simulink model "fmtx_datafm_image_audio"  (R2014b)
settings: Solver=ode45  StartTime=0.0  StopTime=1000*100/3e3  RelTol=1e-3
PreLoadFcn:
  | %%%%%%%%%%%%%%%%%%%%%%%%%%%%%%%%%%%%%%%%%%%%%%%%%%%%%%%%%%%%%%%%%%%%%%%%%%%
  | % check to see if Simulink library folder is missing from the MATLAB path %
  | %%%%%%%%%%%%%%%%%%%%%%%%%%%%%%%%%%%%%%%%%%%%%%%%%%%%%%%%%%%%%%%%%%%%%%%%%%%
  | if isempty(strfind(path, 'rtlsdr_book_library'))
  | 
  |     % create error window
  |     fig_error = figure(...
  |         'Name', 'Error: RTL-SDR Book Library',...
  |         'Toolbar','none',...
  |         'MenuBar','none',...
  |         'NumberTitle','off',...
  |         'Resize','off',...
  |         'WindowStyle','modal');
  |     fig_error.Position(3) = 600;
  |     fig_error.Position(4) = 150;
  |     fig_axes = axes(...
  |         'Parent',fig_error,...
  |         'Position',[0,0,1,1],...
  |         'visible','off');
  |     % error message
  |     t_title = text(.05,.8,...
  |         'MISSING DIRECTORIES',...
  |         'FontSize',11.5);
  |     t_body = text(.075,.6,...
  |         [{'Simulink cannot find the  \it{<root>}\rm / \it{rtlsdr\_book\_library}\rm  folder in the \it{MATLAB Path}\rm.'},...
  |         {'Please set the MATLAB path following the instructions given in Exercise 2.4.'}],...
  |         'FontSize',10.5);
  |     % buttons
  |     btn_path = uicontrol(...
  |         'Parent',fig_error,...
  |         'String','Set Path Now',...
  |         'FontSize',10,...
  |         'Callback', 'pathtool; close(fig_error);',...
  |         'Position', [fig_error.Position(3)/2-210, 30, 200, 30]);
  |     btn_abort = uicontrol(...
  |         'Parent',fig_error,...
  |         'String','No thanks',...
  |         'FontSize',10,...
  |         'Callback', 'close(fig_error); abort=1;',...
  |         'Position', [fig_error.Position(3)/2+10, 30, 200, 30]);
  | 
  |     % pause to allow user to interact with error box
  |     uiwait(fig_error);
  | 
  |     % abort simulation
  |     try
  |         if abort==1
  |             set_param(gcs, 'SimulationCommand', 'stop');
  |         end
  |     end
  | 
  |     % if user has set path, allow diagram to be updated
  |     if ~exist('abort','var')
  |         % create error window
  |         fig_update = figure(...
  |             'Name', 'Update Diagram',...
  |             'Toolbar','none',...
  |             'MenuBar','none',...
  |             'NumberTitle','off',...
  |             'Resize','off');
  |         fig_update.Position(3) = 400;
  |         fig_update.Position(4) = 120;
  |         fig_axes = axes(...
  |             'Parent',fig_update,...
  |             'Position',[0,0,1,1],...
  |             'visible','off');
  |         % instruction message
  |         t_body = text(.075,.7,...
  |             'Once you have set the path, update the block diagram',...
  |             'FontSize',10.5);
  |         % button
  |         btn_update = uicontrol(...
  |             'Parent',fig_update,...
  |             'String','Update Block Diagram',...
  |             'FontSize',10,...
  |             'Callback', 'set_param(gcs,''SimulationCommand'',''update''); close(gcf)',...
  |             'Position', [fig_update.Position(3)/2-100, 30, 200, 30]);
  |     end
  | 
  |     % clear error components
  |     clear('fig_error','fig_update','fig_axes','t_title','t_body','btn_path','btn_abort','btn_update','abort');
  | 
  | end
  | %%%%%%%%%%%%%%%%%%%%%%%%%%%%%%%%%%%%%%%%%%%%%%%%%%%%%%%%%%%%%%%%%%%%%%%%%%%
undefined symbols (not defined in the file): dfilt, fdesignblkfcn, gcbh
libraries: dspvision x2, rtlsdr_book_library x2, dsparch4 x1, dspsrcs4 x1
CloseFcn:
  | closefcn_model;
Description:
  | Software, Simulation Examples and Design Exercises Licence Agreement
  | 
  | This license agreement refers to the simulation examples, design exercises and files,
  | and associated software MATLAB and Simulink resources that accompany the book:
  | 
  |      Title: Software Defined Radio using MATLAB & Simulink and the RTL-SDR
  |      Published by Strathclyde Academic Media, 2015
  |      Authored by Robert W. Stewart, Kenneth W. Barlee, Dale S.W. Atkinson,
  |      and Louise H. Crockett
  | 
  | and made available as a download from, www.desktopSDR.com or variously acquired
  | by other means such as via USB storage, cloud storage, disk or any other electronic
  | or optical or magnetic storage mechanism. These files and associated software may
  | be used subject to the terms of agreement of the conditions below:
  | 
  |     Copyright © 2015 Robert W. Stewart, Kenneth W. Barlee, Dale S.W. Atkinson,
  |     and Louise H. Crockett
  |     All rights reserved.
  | 
  | Redistribution and use in source and binary forms, with or without modification, are
  | permitted provided that the following conditions are met:
  | 
  |    1.  Redistributions of source code must retain the above copyright notice, this list of
  |         conditions and the following disclaimer.
  | 
  |    2.  Redistributions in binary form must reproduce the above copyright notice, this
  |         list of conditions and the following disclaimer in the documentation and/or other
  |         materials provided with the distribution.
  | 
  |    3.  Neither the name of the copyright holder nor the names of its contributors may
  |         be used to endorse or promote products derived from this software without
  |         specific prior written permission.
  | 
  |    4.  In all cases, the software is, and all modifications and derivatives of the
  |         software shall be, licensed to you solely for use in conjunction with The
  |         MathWorks, Inc. products and service offerings.
  | 
  | THIS SOFTWARE IS PROVIDED BY THE COPYRIGHT HOLDERS AND CONTRIBUTORS
  | "AS IS" AND ANY EXPRESS OR IMPLIED WARRANTIES, INCLUDING, BUT NOT LIMITED
  | TO, THE IMPLIED WARRANTIES OF MERCHANTABILITY AND FITNESS FOR A
  | PARTICULAR PURPOSE ARE DISCLAIMED. IN NO EVENT SHALL THE COPYRIGHT
  | HOLDER OR CONTRIBUTORS BE LIABLE FOR ANY DIRECT, INDIRECT, INCIDENTAL,
  | SPECIAL, EXEMPLARY, OR CONSEQUENTIAL DAMAGES (INCLUDING, BUT NOT
  | LIMITED TO, PROCUREMENT OF SUBSTITUTE GOODS OR SERVICES; LOSS OF USE,
  | DATA, OR PROFITS; OR BUSINESS INTERRUPTION) HOWEVER CAUSED AND ON ANY
  | THEORY OF LIABILITY, WHETHER IN CONTRACT, STRICT LIABILITY, OR TORT
  | (INCLUDING NEGLIGENCE OR OTHERWISE) ARISING IN ANY WAY OUT OF THE USE
  | OF THIS SOFTWARE, EVEN IF ADVISED OF THE POSSIBILITY OF SUCH DAMAGE.
  | 
  | 
  | Audio Tracks used in Simulations Examples and Design Exercises
  | 
  | The music and vocal files used within the Examples files and software within the book
  | were variously written, arranged, performed, recorded and produced by Garrey Rice,
  | Adam Struth, Jamie Struth, Iain Thistlethwaite and also Marshall Craigmyle who
  | collectively, and individually where appropriate, assert and retain all of their copyright,
  | performance and artistic rights. Permission to use and reproduce this music is
  | granted for all purposes associated with MATLAB and Simulink software and the
  | simulation examples and design exercises files that accompany this book. Requests to
  | use the music for any other purpose should be directed to: info@desktopSDR.com.
  | For information on music track names, full credits, and links to the musicians please
  | refer to www.desktopSDR.com/more/audio.
settings Model: Creator=desktopSDR Team  LastModifiedBy=desktopSDR Team
settings DataIOCC: LimitDataPoints=off  SaveOutput=off  SignalLogging=off  SaveTime=off

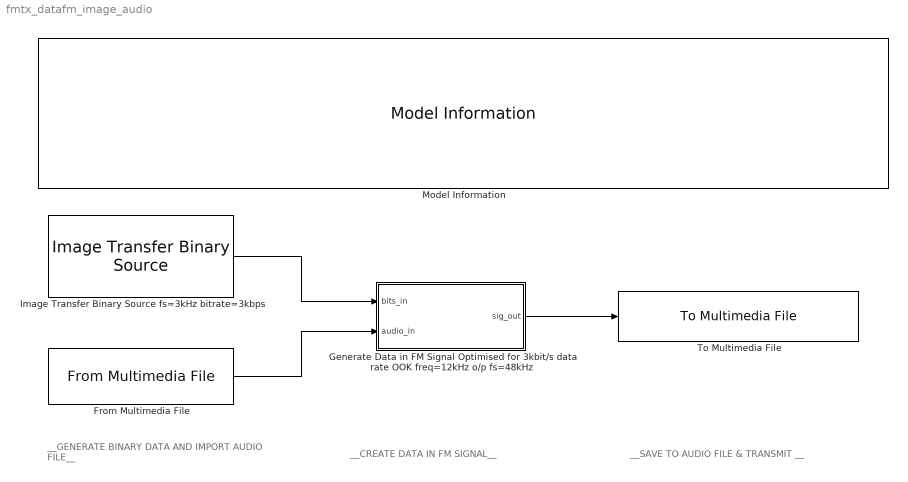
== system fmtx_datafm_image_audio ==
  note: __CREATE DATA IN FM SIGNAL__
  note: __SAVE TO AUDIO FILE & TRANSMIT __
  note: __GENERATE BINARY DATA
      | AND IMPORT AUDIO FILE__
  From Multimedia File : dspvision/From Multimedia File  inputFilename=..\..\audio_sources\music3_mono48kHz.wav  loop=on  numPlays=inf  outputStreams=Audio only  videoDataType=single  audioDataType=double  inheritSampleTime=on  userDefinedSampleTime=1/30  noAudioOutput=off  isIntensityVideo=off  fourcc=RGB  colorVideoFormat=Separate color signals  outputEOF=off  dataOrg=Column-major  audioFrameSize=1024  computeAudioFrameSize=off  outSamplingMode=Frame based
  Generate Data in FM Signal Optimised for 3kbit/s data rate OOK freq=12kHz o/p fs=48kHz : Subsystem
  Image Transfer Binary Source fs=3kHz bitrate=3kbps : rtlsdr_book_library/Data Comms Sources and Sinks/Image Transfer Binary Source  filename=image1.mat  fs=3e3
  Model Information : rtlsdr_book_library/Additional Tools/Model Information/Model Information
  To Multimedia File : dspvision/To Multimedia File  outputFilename=fmtx_datafm_image1_audio.wav  streamSelection=Audio only  videoCompressor=None (uncompressed)  audioCompressor=None (uncompressed)  imagePorts=Separate color signals  fileType=WAV  audioDatatype=16-bit integer  fourcc=RGB  videoQuality=75  mj2000CompFactor=10
  wires:
  Generate Data in FM Signal Optimised for 3kbit/s data rate OOK freq=12kHz o/p fs=48kHz/1(sig_out) -> To Multimedia File/1
  From Multimedia File/1 -> Generate Data in FM Signal Optimised for 3kbit/s data rate OOK freq=12kHz o/p fs=48kHz/2(audio_in)
  Image Transfer Binary Source fs=3kHz bitrate=3kbps/1 -> Generate Data in FM Signal Optimised for 3kbit/s data rate OOK freq=12kHz o/p fs=48kHz/1(bits_in)

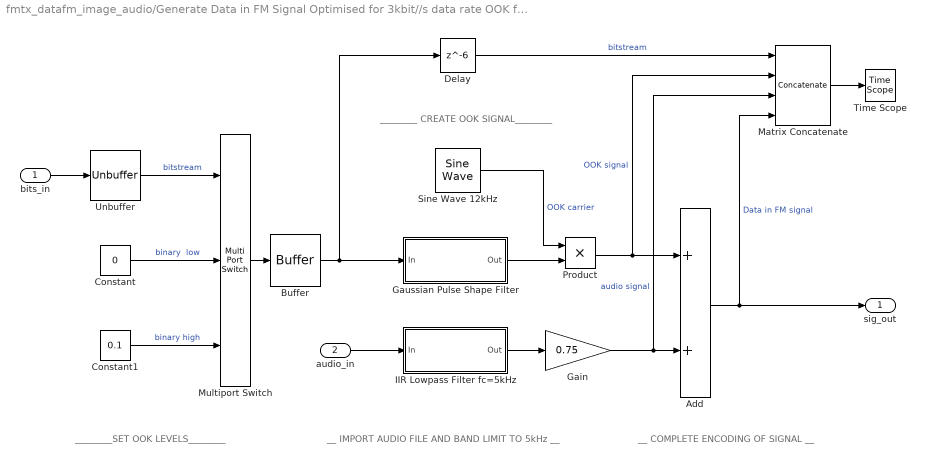
== system fmtx_datafm_image_audio/Generate Data in FM Signal Optimised for 3kbit//s data rate OOK freq=12kHz o//p fs=48kHz ==
  note: __ IMPORT AUDIO FILE AND BAND LIMIT TO 5kHz __
  note: __ COMPLETE ENCODING OF SIGNAL __
  note: ________ CREATE OOK SIGNAL________
  note: ________SET OOK LEVELS________
  bits_in : Inport
  audio_in : Inport  Port=2
  Add : Sum
  Buffer : Buffer  N=1024  TreatMby1Signals=One channel
  Constant : Constant  Value=0  SampleTime=1/48e3
  Constant1 : Constant  Value=0.1  SampleTime=1/48e3
  Delay : Delay  DelayLength=6  InputProcessing=Columns as channels (frame based)
  Gain : Gain  Gain=0.75
  Gaussian Pulse Shape Filter : Subsystem  DialogController=fdesignblkfcn  InitFcn=fdesignblkfcn(gcbh, {'InitFcn'});  mask(Pulse Shaping Filter){}
      mask help: Design a Pulse Shaping Filter
      settings: CopyFcn=fdesignblkfcn(gcbh, {'CopyFcn'});
      mask Help: helpview(mapfilelocation('dsp'), 'dsppulseshapingfilter');
      mask Display: disp('Pulse Shaping');
  IIR Lowpass Filter fc=5kHz : Subsystem  DialogController=fdesignblkfcn  InitFcn=fdesignblkfcn(gcbh, {'InitFcn'});  mask(Lowpass Filter){}
      mask help: Design a lowpass filter
      settings: CopyFcn=fdesignblkfcn(gcbh, {'CopyFcn'});
      mask Help: helpview(mapfilelocation('dsp'), 'dsplowpassfilter');
      mask Display: disp('Lowpass')
  Matrix Concatenate : Concatenate  NumInputs=4  Mode=Multidimensional array  ConcatenateDimension=2
  Multiport Switch : MultiPortSwitch  DataPortOrder=Specify indices  Inputs=2  DataPortIndices={0,1}
  Product : Product
  Sine Wave 12kHz : dspsrcs4/Sine Wave  Amplitude=1  Frequency=12e3  Phase=pi/6  SampleMode=Discrete  OutComplex=Real  CompMethod=Trigonometric fcn  TableSize=Speed  SampleTime=1/48e3  SamplesPerFrame=1024  ResetState=Restart at time zero  dataType=double  wordLen=16  udDataType=sfix(16)  fracBitsMode=Best precision  numFracBits=15  OutDataTypeStr=double  LastOutDataTypeStr=double
  Time Scope : TimeScope  StartFcn=startfcn_time_scope  DefaultConfigurationName=spbscopes.TimeScopeBlockCfg
  Unbuffer : Unbuffer  SampleBasedProcessing=Same as frame based
  sig_out : Outport
  wires:
  bits_in/1 -> Unbuffer/1
  audio_in/1 -> IIR Lowpass Filter fc=5kHz/1(In)
  Constant1/1 -> Multiport Switch/3  "binary high"
  Constant/1 -> Multiport Switch/2  "binary  low"
  Matrix Concatenate/1 -> Time Scope/1
  IIR Lowpass Filter fc=5kHz/1(Out) -> Gain/1
  Gain/1 -> Matrix Concatenate/3, Add/2  "audio signal"
  Unbuffer/1 -> Multiport Switch/1  "bitstream"
  Sine Wave 12kHz/1 -> Product/1  "OOK carrier"
  Buffer/1 -> Delay/1, Gaussian Pulse Shape Filter/1(In)
  Gaussian Pulse Shape Filter/1(Out) -> Product/2
  Product/1 -> Matrix Concatenate/2, Add/1  "OOK signal"
  Multiport Switch/1 -> Buffer/1
  Add/1 -> Matrix Concatenate/4, sig_out/1  "Data in FM signal"
  Delay/1 -> Matrix Concatenate/1  "bitstream"

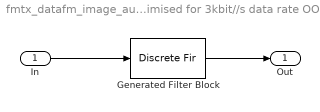
== system fmtx_datafm_image_audio/Generate Data in FM Signal Optimised for 3kbit//s data rate OOK freq=12kHz o//p fs=48kHz/Gaussian Pulse Shape Filter ==
  In : Inport
  Generated Filter Block : DiscreteFir  Tag=BlockMethodSubSystem  Coefficients=[0.011762699801536648 0.02574058949880206 0.048853030996808648 0.080412967456829659 0.11479479958541473 0.14212808000788887 0.15261566530543869 0.14212808000788887 0.11479479958541473 0.080412967456829659 0.048853030996808648 0.02574058949880206 0.011762699801536648]  InputProcessing=Columns as channels (frame based)
  Out : Outport
  wires:
  In/1 -> Generated Filter Block/1
  Generated Filter Block/1 -> Out/1

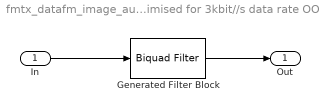
== system fmtx_datafm_image_audio/Generate Data in FM Signal Optimised for 3kbit//s data rate OOK freq=12kHz o//p fs=48kHz/IIR Lowpass Filter fc=5kHz ==
  In : Inport
  Generated Filter Block : dsparch4/Biquad Filter  Tag=BlockMethodSubSystem  IIRFiltStruct=Direct form II  CoeffSource=Specify via dialog  BiQuadCoeffs=[0.042969561565618077 0.085939123131236153 0.042969561565618077 1 -1.555657758639478 0.87862894950711246;0.061935778665187145 0.12387155733037429 0.061935778665187145 1 -1.4205854439157277 0.71551417743867618;0.076267506257963871 0.15253501251592774 0.076267506257963871 1 -1.3129466799361755 0.58552845469333503;0.086601072542009133 0.17320214508401827 0.086601072542009133 1 -1.2285300304649582 0.48358600582481348;0.093330556989539987 0.18666111397907997 0.093330556989539987 1 -1.163928907888546 0.40557299919227274;0.096444753467057845 0.19288950693411569 0.096444753467057845 1 -1.1165183760349042 0.34831953379659664;0.093941235402774201 0.1878824708055484 0.093941235402774201 1 -1.0843804969696778 0.30950948727293498;0.06178520401543218 0.12357040803086436 0.06178520401543218 1 -1.0662257647565232 0.28758563845929269;0.055723392794766298 0.1114467855895326 0.055723392794766298 1 -1.0621451972418323 0.28265790148054942;0.057022086237706486 0.11404417247541297 0.057022086237706486 1 -1.0736131368995174 0.29650670807858259;0.059076157735379158 0.11815231547075832 0.059076157735379158 1 -1.0986348427077246 0.32672318765855057;0.061968373960671889 0.12393674792134378 0.061968373960671889 1 -1.1382102890943879 0.37451492003590464;0.065816095114757556 0.13163219022951511 0.065816095114757556 1 -1.1939341274770339 0.44180762331972157;0.070775447994568252 0.1415508959891365 0.070775447994568252 1 -1.2680675169023181 0.53133189736134834;0.077044306786640995 0.15408861357328199 0.077044306786640995 1 -1.3636185258276994 0.64672031780597239;0.027416633436479335 0.054833266872958669 0.027416633436479335 1 -1.4843995625697666 0.79257678971633061;0.025182438141471038 0.050364876282942075 0.025182438141471038 1 -1.6349915970637752 0.97443334138682025;0.04855389746467715 0.097107794929354299 0.04855389746467715 1 -1.5190593292115486 0.83443229465294233;0.067085454415403187 0.13417090883080637 0.067085454415403187 1 -1.3912817200511742 0.68012668705103563;0.081497123248148048 0.1629942464962961 0.081497123248148048 1 -1.2898124076148489 0.55759125998115422;0.092395363974827269 0.18479072794965454 0.092395363974827269 1 -1.210637439466447 0.46197872154598202;0.10020909151780877 0.20041818303561754 0.10020909151780877 1 -1.1505510212366299 0.38941772017415877;0.10527662371649776 0.21055324743299553 0.10527662371649776 1 -1.1071126518721077 0.33696108068878605;0.10764709070254799 0.21529418140509599 0.10764709070254799 1 -1.0785684378951543 0.30249078256554834;0.061743519146292225 0.12348703829258445 0.061743519146292225 1 -1.0637754129904147 0.28462656745622505;0.055510029644634425 0.11102005928926885 0.055510029644634425 1 -1.061331093635125 0.28167478125698797;0.056629126444816269 0.11325825288963254 0.056629126444816269 1 -1.0695023053542168 0.29154242393275437;0.058487856243194969 0.11697571248638994 0.058487856243194969 1 -1.0910637531749297 0.31758025895419473;0.06116095659595399 0.12232191319190798 0.06116095659595399 1 -1.1268755842462319 0.36082700921901179;0.064756747550877514 0.12951349510175503 0.064756747550877514 1 -1.1783777543589316 0.42302158074274743;0.069421296340545946 0.13884259268109189 0.069421296340545946 1 -1.2476572474610272 0.50668423766453741;0.075341935222395684 0.15068387044479137 0.075341935222395684 1 -1.3375283160935707 0.61521350145575437;0.076281548564130483 0.15256309712826097 0.076281548564130483 1 -1.4516002590171362 0.75296799990671892;0.27118984696313492 0.54237969392626983 0.27118984696313492 1 -1.5942748095188128 0.92526331321828925]  a0Flag=Warning  IC=0  ICnum=0  ICden=0  InputProcessing=Columns as channels (frame based)  denAccumFracLength=30  denProdOutputFracLength=30  secondMemoryFracLength=15  roundingMode=Floor  overflowMode=off  ScaleValues=[0.067729897263719196;1;1;1;1;1;1;1;1;1;1;1;1;1;1;1;1;1;1;1;1;1;1;1;1;1;1;1;1;1;1;1;1;1;1]  optimizeScaleValues=off  ScaleValueMode=Specify via input port (g)  scaleValueFracLength=14  FilterSource=Specify via dialog  dfiltObjectName=dfilt.df2tsos([1 0.3 0.4],[1 0.1 0.2])
  Out : Outport
  wires:
  In/1 -> Generated Filter Block/1
  Generated Filter Block/1 -> Out/1
